simulink model "IMUsensor"  (R2023b)
settings: Solver=VariableStepAuto  StartTime=0.0  StopTime=10.0  RelTol=1e-3
settings Model: Creator=user  LastModifiedBy=user

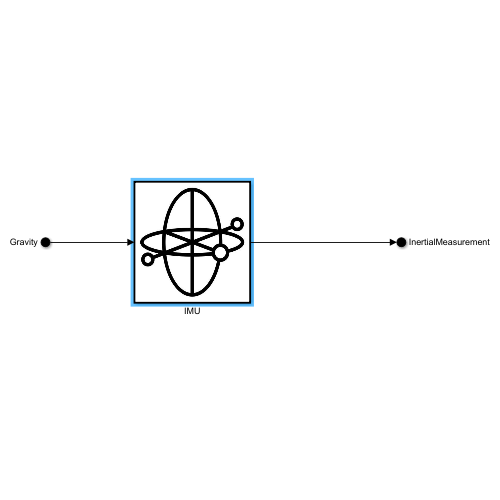
[thumbnail: Simulink's stored preview of the top-level diagram]
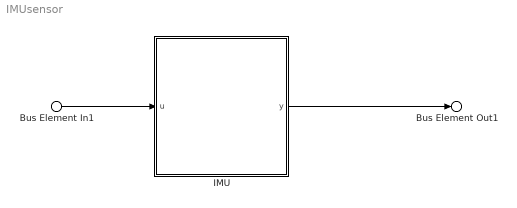
== system IMUsensor ==
  Bus Element In1 : Inport  PortName=Gravity
  IMU : MATLAB Function  TreatAsAtomicUnit=on
  Bus Element Out1 : Outport  PortName=InertialMeasurement
  wires:
  Bus Element In1/1 -> IMU/1(u)
  IMU/1(y) -> Bus Element Out1/1

== matlab function IMUsensor/IMU ==
  data: u input; y output
function y = fcn(u)

u = [0.12; 2; 0.003; 0.3; 0.62; 2.3];

y = u;
